simulink library "lib_header_20a"  (R2020a)
settings: Solver=VariableStepAuto  StartTime=0.0  StopTime=10.0  RelTol=1e-3
undefined symbols (not defined in the file): fs
libraries: xpcutilitieslib x1
settings Model: Creator=jiw19031  LastModifiedBy=mrajase
settings DebuggingCC: SFMachineParentedDataDiag=error

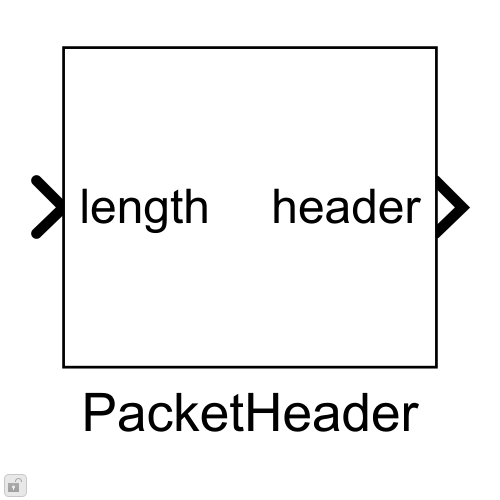
[thumbnail: Simulink's stored preview of the top-level diagram]
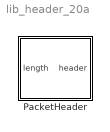
== system lib_header_20a ==
  PacketHeader : Subsystem  mask{src=0, dst=0, pkt_type=0, pkt_priority=0, service=0, flag=0, option1=0, option2=0, subframe_num=0}
      mask prompts: pkt_type "Type"; pkt_priority "Priority"; subframe_num "SubframeNum"

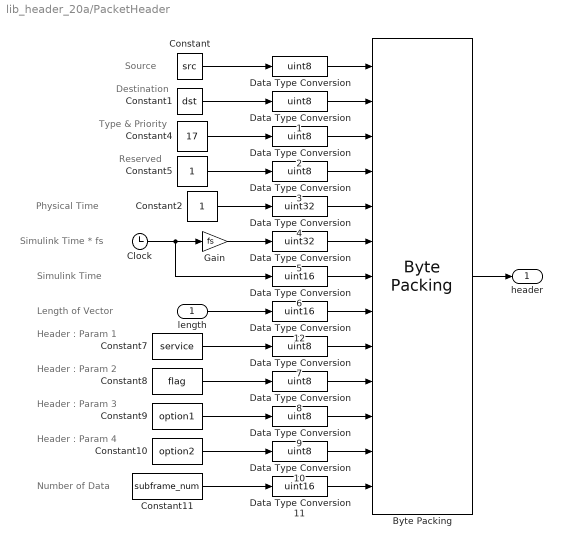
== system lib_header_20a/PacketHeader ==
  note: Source
  note: Destination
  note: Type & Priority
  note: Reserved
  note: Physical Time
  note: Simulink Time * fs
  note: Simulink Time
  note: Length of Vector
  note: Header : Param 1
  note: Header : Param 2
  note: Header : Param 3
  note: Header : Param 4
  note: Number of Data
  length : Inport
  "Byte Packing " : xpcutilitieslib/Byte Packing   MaskPackedDataType=uint8  MaskUnpackedDataTypes={'uint8','uint8','uint8','uint8','uint32','uint32','uint16','uint16','uint8','uint8','uint8','uint8','uint16'}  MaskAlignment=1
  Clock : Clock
  Constant : Constant  Value=src
  Constant1 : Constant  Value=dst
  Constant10 : Constant  Value=option2
  Constant11 : Constant  Value=subframe_num
  Constant2 : Constant
  Constant4 : Constant  Value=17
  Constant5 : Constant
  Constant7 : Constant  Value=service
  Constant8 : Constant  Value=flag
  Constant9 : Constant  Value=option1
  Data Type Conversion{,1..3,7..10} (8 alike) : DataTypeConversion  OutDataTypeStr=uint8
  Data Type Conversion11 : DataTypeConversion  OutDataTypeStr=uint16
  Data Type Conversion12 : DataTypeConversion  OutDataTypeStr=uint16
  Data Type Conversion4 : DataTypeConversion  OutDataTypeStr=uint32
  Data Type Conversion5 : DataTypeConversion  OutDataTypeStr=uint32
  Data Type Conversion6 : DataTypeConversion  OutDataTypeStr=uint16
  Gain : Gain  Gain=fs
  header : Outport
  wires:
  "Byte Packing "/1 -> header/1
  length/1 -> Data Type Conversion12/1
  Constant/1 -> Data Type Conversion/1
  Constant1/1 -> Data Type Conversion1/1
  Constant4/1 -> Data Type Conversion2/1
  Constant5/1 -> Data Type Conversion3/1
  Constant2/1 -> Data Type Conversion4/1
  Constant7/1 -> Data Type Conversion7/1
  Constant8/1 -> Data Type Conversion8/1
  Constant9/1 -> Data Type Conversion9/1
  Constant10/1 -> Data Type Conversion10/1
  Constant11/1 -> Data Type Conversion11/1
  Gain/1 -> Data Type Conversion5/1
  Clock/1 -> Data Type Conversion6/1, Gain/1
  Data Type Conversion/1 -> "Byte Packing "/1
  Data Type Conversion1/1 -> "Byte Packing "/2
  Data Type Conversion2/1 -> "Byte Packing "/3
  Data Type Conversion3/1 -> "Byte Packing "/4
  Data Type Conversion4/1 -> "Byte Packing "/5
  Data Type Conversion5/1 -> "Byte Packing "/6
  Data Type Conversion6/1 -> "Byte Packing "/7
  Data Type Conversion12/1 -> "Byte Packing "/8
  Data Type Conversion7/1 -> "Byte Packing "/9
  Data Type Conversion8/1 -> "Byte Packing "/10
  Data Type Conversion9/1 -> "Byte Packing "/11
  Data Type Conversion10/1 -> "Byte Packing "/12
  Data Type Conversion11/1 -> "Byte Packing "/13
